simulink model "SimulationCarTC1"  (Simulink 8.8)
settings: Solver=FixedStepAuto  StartTime=0.0  StopTime=10.0  RelTol=1e-3
model workspace: external: MAT-File C:\Users\EMIdev1\Documents\GitHub\DRI001-MPS-2018.2.3-601-2\DRI006\DRIPSamples\CollisionWarningSystem\external\SlkModels\SimulationCarTC1.mat (data not in the file)
undefined symbols (not defined in the file or in its folder): detectionRange, driverReacionTime, frictionCoef, subjectPosition, subjectVelocity, targetPosition, targetVelocity
(part 2 of 2)

== system SimulationCarTC1/Assert/Assert_1/existsAndStay/universally/from ==
  instTrue : Inport
  Constant1 : Constant  Value=0  OutDataTypeStr=uint8
      settings: AttributesFormatString=%<Description>
  Data Type Conversion : DataTypeConversion  OutDataTypeStr=uint8
  Memory : Memory
  Relational Operator2 : RelationalOperator  Operator=>  OutDataTypeStr=boolean  RndMeth=Nearest
  Sum1 : Sum  Inputs=|++
  avoidOverflow : Subsystem
  qualifierTrue : Outport
  wires:
  avoidOverflow/1(Out) -> Sum1/2
  Data Type Conversion/1 -> Sum1/1
  Relational Operator2/1 -> qualifierTrue/1
  instTrue/1 -> Data Type Conversion/1
  Constant1/1 -> Relational Operator2/2
  Sum1/1 -> Relational Operator2/1, Memory/1
  Memory/1 -> avoidOverflow/1(In)

== system SimulationCarTC1/Constraint/Constraint_1/universally/from/avoidOverflow ==
  In : Inport
  Constant : Constant  Value=100
  Constant1 : Constant
  Relational Operator : RelationalOperator  Operator=<  OutDataTypeStr=boolean  RndMeth=Nearest
  Switch : Switch  Criteria=u2 > Threshold  Threshold=0.5
  Out : Outport
  wires:
  Switch/1 -> Out/1
  Constant1/1 -> Switch/3
  Constant/1 -> Relational Operator/2
  In/1 -> Relational Operator/1, Switch/1
  Relational Operator/1 -> Switch/2

== system SimulationCarTC1/Constraint/Constraint_1_cond/betweenOC/after/avoidOverflow ==
  In : Inport
  Constant : Constant  Value=100
  Constant1 : Constant
  Relational Operator : RelationalOperator  Operator=<  OutDataTypeStr=boolean  RndMeth=Nearest
  Switch : Switch  Criteria=u2 > Threshold  Threshold=0.5
  Out : Outport
  wires:
  Switch/1 -> Out/1
  Constant1/1 -> Switch/3
  Constant/1 -> Relational Operator/2
  In/1 -> Relational Operator/1, Switch/1
  Relational Operator/1 -> Switch/2

== system SimulationCarTC1/Constraint/Constraint_1_cond/betweenOC/until/avoidOverflow ==
  In : Inport
  Constant : Constant  Value=100
  Constant1 : Constant
  Relational Operator : RelationalOperator  Operator=<  OutDataTypeStr=boolean  RndMeth=Nearest
  Switch : Switch  Criteria=u2 > Threshold  Threshold=0.5
  Out : Outport
  wires:
  Switch/1 -> Out/1
  Constant1/1 -> Switch/3
  Constant/1 -> Relational Operator/2
  In/1 -> Relational Operator/1, Switch/1
  Relational Operator/1 -> Switch/2

== system SimulationCarTC1/Constraint/Constraint_1_cond/existsAndStay/universally/from ==
  instTrue : Inport
  Constant1 : Constant  Value=0  OutDataTypeStr=uint8
      settings: AttributesFormatString=%<Description>
  Data Type Conversion : DataTypeConversion  OutDataTypeStr=uint8
  Memory : Memory
  Relational Operator2 : RelationalOperator  Operator=>  OutDataTypeStr=boolean  RndMeth=Nearest
  Sum1 : Sum  Inputs=|++
  avoidOverflow : Subsystem
  qualifierTrue : Outport
  wires:
  avoidOverflow/1(Out) -> Sum1/2
  Data Type Conversion/1 -> Sum1/1
  Relational Operator2/1 -> qualifierTrue/1
  instTrue/1 -> Data Type Conversion/1
  Constant1/1 -> Relational Operator2/2
  Sum1/1 -> Relational Operator2/1, Memory/1
  Memory/1 -> avoidOverflow/1(In)

== system SimulationCarTC1/Highlevel/Highlevel_1/universally/from/avoidOverflow ==
  In : Inport
  Constant : Constant  Value=100
  Constant1 : Constant
  Relational Operator : RelationalOperator  Operator=<  OutDataTypeStr=boolean  RndMeth=Nearest
  Switch : Switch  Criteria=u2 > Threshold  Threshold=0.5
  Out : Outport
  wires:
  Switch/1 -> Out/1
  Constant1/1 -> Switch/3
  Constant/1 -> Relational Operator/2
  In/1 -> Relational Operator/1, Switch/1
  Relational Operator/1 -> Switch/2

== system SimulationCarTC1/Highlevel/Highlevel_10/universally/from/avoidOverflow ==
  In : Inport
  Constant : Constant  Value=100
  Constant1 : Constant
  Relational Operator : RelationalOperator  Operator=<  OutDataTypeStr=boolean  RndMeth=Nearest
  Switch : Switch  Criteria=u2 > Threshold  Threshold=0.5
  Out : Outport
  wires:
  Switch/1 -> Out/1
  Constant1/1 -> Switch/3
  Constant/1 -> Relational Operator/2
  In/1 -> Relational Operator/1, Switch/1
  Relational Operator/1 -> Switch/2

== system SimulationCarTC1/Highlevel/Highlevel_11/universally/from/avoidOverflow ==
  In : Inport
  Constant : Constant  Value=100
  Constant1 : Constant
  Relational Operator : RelationalOperator  Operator=<  OutDataTypeStr=boolean  RndMeth=Nearest
  Switch : Switch  Criteria=u2 > Threshold  Threshold=0.5
  Out : Outport
  wires:
  Switch/1 -> Out/1
  Constant1/1 -> Switch/3
  Constant/1 -> Relational Operator/2
  In/1 -> Relational Operator/1, Switch/1
  Relational Operator/1 -> Switch/2

== system SimulationCarTC1/Highlevel/Highlevel_12/universally/from/avoidOverflow ==
  In : Inport
  Constant : Constant  Value=100
  Constant1 : Constant
  Relational Operator : RelationalOperator  Operator=<  OutDataTypeStr=boolean  RndMeth=Nearest
  Switch : Switch  Criteria=u2 > Threshold  Threshold=0.5
  Out : Outport
  wires:
  Switch/1 -> Out/1
  Constant1/1 -> Switch/3
  Constant/1 -> Relational Operator/2
  In/1 -> Relational Operator/1, Switch/1
  Relational Operator/1 -> Switch/2

== system SimulationCarTC1/Highlevel/Highlevel_13/universally/from/avoidOverflow ==
  In : Inport
  Constant : Constant  Value=100
  Constant1 : Constant
  Relational Operator : RelationalOperator  Operator=<  OutDataTypeStr=boolean  RndMeth=Nearest
  Switch : Switch  Criteria=u2 > Threshold  Threshold=0.5
  Out : Outport
  wires:
  Switch/1 -> Out/1
  Constant1/1 -> Switch/3
  Constant/1 -> Relational Operator/2
  In/1 -> Relational Operator/1, Switch/1
  Relational Operator/1 -> Switch/2

== system SimulationCarTC1/Highlevel/Highlevel_3/universally/from/avoidOverflow ==
  In : Inport
  Constant : Constant  Value=100
  Constant1 : Constant
  Relational Operator : RelationalOperator  Operator=<  OutDataTypeStr=boolean  RndMeth=Nearest
  Switch : Switch  Criteria=u2 > Threshold  Threshold=0.5
  Out : Outport
  wires:
  Switch/1 -> Out/1
  Constant1/1 -> Switch/3
  Constant/1 -> Relational Operator/2
  In/1 -> Relational Operator/1, Switch/1
  Relational Operator/1 -> Switch/2

== system SimulationCarTC1/Highlevel/Highlevel_4/universally/from/avoidOverflow ==
  In : Inport
  Constant : Constant  Value=100
  Constant1 : Constant
  Relational Operator : RelationalOperator  Operator=<  OutDataTypeStr=boolean  RndMeth=Nearest
  Switch : Switch  Criteria=u2 > Threshold  Threshold=0.5
  Out : Outport
  wires:
  Switch/1 -> Out/1
  Constant1/1 -> Switch/3
  Constant/1 -> Relational Operator/2
  In/1 -> Relational Operator/1, Switch/1
  Relational Operator/1 -> Switch/2

== system SimulationCarTC1/Highlevel/Highlevel_6/universally/from/avoidOverflow ==
  In : Inport
  Constant : Constant  Value=100
  Constant1 : Constant
  Relational Operator : RelationalOperator  Operator=<  OutDataTypeStr=boolean  RndMeth=Nearest
  Switch : Switch  Criteria=u2 > Threshold  Threshold=0.5
  Out : Outport
  wires:
  Switch/1 -> Out/1
  Constant1/1 -> Switch/3
  Constant/1 -> Relational Operator/2
  In/1 -> Relational Operator/1, Switch/1
  Relational Operator/1 -> Switch/2

== system SimulationCarTC1/Highlevel/Highlevel_7/universally/from/avoidOverflow ==
  In : Inport
  Constant : Constant  Value=100
  Constant1 : Constant
  Relational Operator : RelationalOperator  Operator=<  OutDataTypeStr=boolean  RndMeth=Nearest
  Switch : Switch  Criteria=u2 > Threshold  Threshold=0.5
  Out : Outport
  wires:
  Switch/1 -> Out/1
  Constant1/1 -> Switch/3
  Constant/1 -> Relational Operator/2
  In/1 -> Relational Operator/1, Switch/1
  Relational Operator/1 -> Switch/2

== system SimulationCarTC1/Assert/Assert_1/existsAndStay/universally/from/avoidOverflow ==
  In : Inport
  Constant : Constant  Value=100
  Constant1 : Constant
  Relational Operator : RelationalOperator  Operator=<  OutDataTypeStr=boolean  RndMeth=Nearest
  Switch : Switch  Criteria=u2 > Threshold  Threshold=0.5
  Out : Outport
  wires:
  Relational Operator/1 -> Switch/2
  In/1 -> Switch/1, Relational Operator/1
  Constant/1 -> Relational Operator/2
  Constant1/1 -> Switch/3
  Switch/1 -> Out/1

== system SimulationCarTC1/Constraint/Constraint_1_cond/existsAndStay/universally/from/avoidOverflow ==
  In : Inport
  Constant : Constant  Value=100
  Constant1 : Constant
  Relational Operator : RelationalOperator  Operator=<  OutDataTypeStr=boolean  RndMeth=Nearest
  Switch : Switch  Criteria=u2 > Threshold  Threshold=0.5
  Out : Outport
  wires:
  Relational Operator/1 -> Switch/2
  In/1 -> Switch/1, Relational Operator/1
  Constant/1 -> Relational Operator/2
  Constant1/1 -> Switch/3
  Switch/1 -> Out/1

== stateflow chart Constraint/Constraint_1_cond/EndpointAtConditionTime_1_1/detectEventTime ==
  state negative
    entry: isTrue = 0;
  state positive
    entry: eventTime = clk; isTrue = 1;
    during: elapsedTime = clk - eventTime;
  state init
    entry: eventTime = init;
  (default) -> init
  init -> positive [order 2] : [inVal > 0.5]
  init -> negative [order 1] : [inVal < 0.5]
  negative -> positive : [inVal > 0.5]
  data: clk input double; elapsedTime output double; eventTime output double; inVal input double; isTrue output double; init input double

== stateflow chart Scenario/Scenario ==
  state Subject [parallel]
    entry: pressPedalsubjectBra = 0;
    settings: executionOrder=1
    state step_1
      entry: subjectThrottle = pressPedal();
    state step_2
      entry: step_2_stpClk = clk;
    state step_3
      entry: subjectThrottle = releasePedal();
      entry: subjectBrake = pressPedal();
      entry: pressPedalsubjectBra = 1;
    (default) -> Subject.step_1
    Subject.step_1 -> Subject.step_2 : [obstacleDetection]
    Subject.step_2 -> step_3 : [(clk - step_2_stpClk) > (driverReacionTime)]
  state Target [parallel]
    settings: executionOrder=2
    state step_1
      entry: targetThrottle = pressPedal();
    state step_2
      entry: targetBrake = pressPedal();
      entry: targetThrottle = releasePedal();
    (default) -> Target.step_1
    Target.step_1 -> Target.step_2 : [(clk) > (5)]
  data: clk input double; obstacleDetection input double; subjectBrake output double; subjectThrottle output double; targetBrake output double; targetThrottle output double; pressPedalsubjectBra output double; driverReacionTime parameter double; step_2_stpClk local double
